simulink model "n2k_parsing"  (Simulink 7.5)
settings: Solver=FixedStepDiscrete  SolverMode=SingleTasking  StartTime=0.0  StopTime=10.0  FixedStep=0.01  RelTol=1e-3
undefined symbols (not defined in the file): enqueueNumberText, Init_Reset, initCommunications
libraries: dsPICdrivers x6, simulink x2, ecan_dspic x1
settings Model: Creator=Bryant  LastModifiedBy=Bryant
settings OptimizationCC: InlineParams=on  OptimizeModelRefInitCode=on  LifeSpan=1
settings HardwareCC: ProdBitPerInt=16  ProdEndianess=LittleEndian  ProdWordSize=16  ProdHWDeviceType=16-bit Generic
settings RTWCC: SystemTargetFile=dspic.tlc  MakeCommand=make_CreateMPLAB  TemplateMakefile=dspic_pic30_gcc.tmf  PostCodeGenCommand=dsPIC_Compile()  Description=Embedded Target for Microchip dsPIC (real-time)  ProcessScript=dspic_make_rtw_hook
settings RTWCC: CustomSource=|
  | ../../../../../ECAN_dspic/circBuffer.c
  | ../../../../../ECAN_dspic/ecanFunctions.c
  | ../../clib/uart2.c
  | extra.c
settings CodeAppCC: IgnoreCustomStorageClasses=off
settings STFCustomTargetCC: IncludeMdlTerminateFcn=off  CombineOutputUpdateFcns=on  SuppressErrorStatus=on  ERTCustomFileBanners=on  SupportContinuousTime=off  SupportNonInlinedSFcns=off  SystemTargetFile=dspic.tlc
settings ERTTargetCC: MultiwordLength=2048  ParMdlRefBuildCompliant=off  CompOptLevelCompliant=off  IncludeMdlTerminateFcn=off  SuppressErrorStatus=on  ERTFirstTimeCompliant=off  ModelStepFunctionPrototypeControlCompliant=off  CPPClassGenCompliant=off  ExtModeMexFile=ext_serial_win32_comm  InlinedParameterPlacement=NonHierarchical  ERTSrcFileBannerTemplate=dsPIC_code_template.cgt  ERTHdrFileBannerTemplate=dsPIC_code_template.cgt  ERTDataSrcFileTemplate=dsPIC_code_template.cgt  ERTDataHdrFileTemplate=dsPIC_code_template.cgt  ERTCustomFileTemplate=dsPIC_main.tlc  ConvertIfToSwitch=off
settings CustomProperty: DataType=string  Value=C:\PROGRA~1\MATLAB\R2010a\bin\win64\gmake

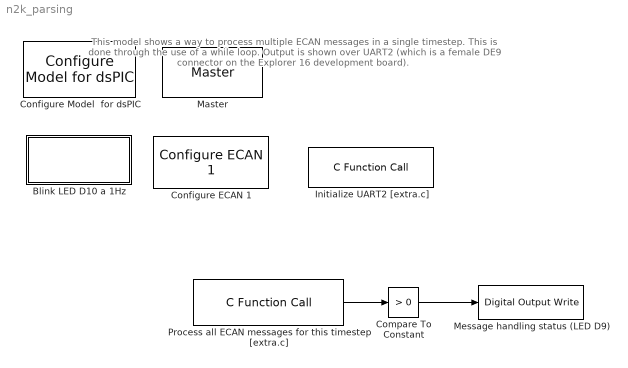
== system n2k_parsing ==
  note: This model shows a way to process multiple ECAN messages in a single timestep. This is done through the use of a while loop.
      | Output is shown over UART2 (which is a female DE9 connector on the Explorer 16 development board).
  Blink LED D10 a 1Hz : Subsystem
      mask Display: disp('blink');
  Compare To Constant : simulink/Logic and Bit Operations/Compare To Constant  SystemSampleTime=-1  relop=>  const=0  LogicOutDataTypeMode=boolean
  Configure ECAN 1 : ecan_dspic/Configure ECAN 1  SystemSampleTime=-1  frame_setting=on  mode=Normal  dma_rx_chan=2  dma_tx_chan=0  baud=250000  ps1=8  pd=5  ps2=6  sjw=4  tq=20  triple_sample=on  dma_buf_size=4 buffers  rx_bufs=[1]  tx_bufs=[0]  buf_0_tx_pri=Highest  buf_0_rte=No  buf_1_tx_pri=Highest  buf_1_rte=No  buf_2_tx_pri=Lowest  buf_2_rte=No  buf_3_tx_pri=Lowest  buf_3_rte=No  buf_4_tx_pri=Lowest  buf_4_rte=No  buf_5_tx_pri=Lowest  buf_5_rte=No  buf_6_tx_pri=Lowest  buf_6_rte=No  buf_7_tx_pri=Lowest  buf_7_rte=No  mask_0=0  mask_0_mide=Match std or ext  mask_1=0  mask_1_mide=Match std or ext  mask_2=0  mask_2_mide=Match std or ext  filters=[0]  filter_0=0  filter_0_mask=0  filter_0_exide=Match only extended  filter_0_buf=1  filter_1=hex2dec('401')  filter_1_mask=0  filter_1_exide=Match only standard  filter_1_buf=2  filter_2=hex2dec('402')  filter_2_mask=0  filter_2_exide=Match only standard  filter_2_buf=3  filter_3=0  filter_3_mask=0  filter_3_exide=Match only standard  filter_3_buf=0  filter_4=0  filter_4_mask=0  filter_4_exide=Match only standard  filter_4_buf=0  filter_5=0  filter_5_mask=0  filter_5_exide=Match only standard  filter_5_buf=0  filter_6=0  filter_6_mask=0  filter_6_exide=Match only standard  filter_6_buf=0  filter_7=0  filter_7_mask=0  filter_7_exide=Match only standard  filter_7_buf=0  filter_8=0  filter_8_mask=0  filter_8_exide=Match only standard  filter_8_buf=0  filter_9=0  filter_9_mask=<empty>  filter_9_exide=Match only standard  filter_9_buf=0  filter_10=0  filter_10_mask=0  filter_10_exide=Match only standard  filter_10_buf=0  filter_11=0  filter_11_mask=0  filter_11_exide=Match only standard  filter_11_buf=0  filter_12=0  filter_12_mask=0  filter_12_exide=Match only standard  filter_12_buf=0  filter_13=0  filter_13_mask=0  filter_13_exide=Match only standard  filter_13_buf=0  filter_14=0  filter_14_mask=0  filter_14_exide=Match only standard  filter_14_buf=0  filter_15=0  filter_15_mask=0  filter_15_exide=Match only standard  filter_15_buf=0
  Configure Model  for dsPIC : dsPICdrivers/Simulink Configuration/Configure Model  for dsPIC
  Initialize UART2 [extra.c] : dsPICdrivers/OTHERS/C Function Call  Tag=dsPIC_dsPIC_CFunctionCall  FctUpdate=None  fctName=enqueueNumberText  INPUT_SIZE=1  INPUT1=uint32  INPUT2=--  INPUT3=--  OUTPUT_SIZE=1  OUTPUT1=--  SampleTime=-1  InputType=[]  OutputType=[]  FctDeclaration=extern void enqueueNumberText();  FctCall=enqueueNumberText();  OrderingInOutPopup=None  FctStart=Start Function (Call once and only once)  FctStart_Name=initCommunications  FctStart_Declaration=inline extern void initCommunications();  FctStart_Call=initCommunications();  FctInit=None  FctInit_Name=Init_Reset  FctInit_Declaration=inline extern void Init_Reset();  FctInit_Call=Init_Reset();  PinDigitalInput=[]  PinDigitalOutput=[]  AnalogueInput=[]
  Master : dsPICdrivers/Master  Tag=dsPIC_MASTER  Priority=1  TimeStepType=Timer1  picType=33fJ256GP710  fcy=40000000  Quartz_33f=8e6  PLLActive_33f=on  fcyDesired_33f=40000000  tmr1="[8  49999  0]"  tmr1Info="Time Step : 0.01  ;   Error : 0%  PR1=49999"  tmr2345="[0  0  0  0  0  0  0  0]"  tmr2345cfg=[-1 -1 -1 -1 -1 -1 -1 -1]  IOautoConf=on  typePort="[ 0   0   0   0   0   0  10  10   0   0   0   0   0   0   0   0   0   0   0   0   0   0   0   0   0   0   0   0   0   0   0   0   0   0   0   0   0   0   0   0   0   0   0   0   0   0   0   0   0   0   0   0   0   0   0   0   0   0   0   0   0   0   0   0   0   0   0   0   0   0   0   0   0   0   0   0   0   0   0   0   0   0   0   0   0   0   0   0   0   0   0   0   0   0   0   0   0   0   0   0   0   0   0   0   0   0   0   0   0   0   0   0 ]"  TRIS="[ 65343  65535  65535  65535  65535  65535  65535 ]"  ADPCFG=12582912  MasterBusyPort=None  MasterOverloadPort=None  FOSC=Quartz (XT - HS)  ClockSwitchMonitor=Both disabled  TempProtection_33f=TEMP_ON  FPBOR=<empty>  PWRT=disable  MCLR=<empty>  ICD=ICS_PGD1  JTAGEN=JTAGEN_OFF  PowerSave=off  OverrideFcy=off  NewFcy=1e6  PR2345="[65535  65535  65535  65535  65535  65535  65535  65535]"
  Message handling status (LED D9) : dsPICdrivers/Digital I//O/Digital Output Write  Tag=dsPIC_Digital_Output  Priority=5  PORT=A  Pin=[6]  Simultaneous=off  OrderingInOutPopup=None
  Process all ECAN messages for this timestep [extra.c] : dsPICdrivers/OTHERS/C Function Call  Tag=dsPIC_dsPIC_CFunctionCall  FctUpdate=Output Function  fctName=processAllMessages  INPUT_SIZE=1  INPUT1=--  INPUT2=--  INPUT3=--  OUTPUT_SIZE=1  OUTPUT1=uint8  SampleTime=.01  InputType=[ ]  OutputType=[ 2 ]  FctDeclaration=extern uint8_T processAllMessages();  FctCall=%y1 = processAllMessages();  OrderingInOutPopup=None  FctStart=None  FctStart_Declaration=inline extern void ();  FctStart_Call=();  FctInit=None  FctInit_Name=Init_Reset  FctInit_Declaration=inline extern void Init_Reset();  FctInit_Call=Init_Reset();  PinDigitalInput=[]  PinDigitalOutput=[]  AnalogueInput=[]
  wires:
  Process all ECAN messages for this timestep [extra.c]/1 -> Compare To Constant/1
  Compare To Constant/1 -> Message handling status (LED D9)/1

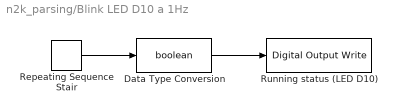
== system n2k_parsing/Blink LED D10 a 1Hz ==
  Data Type Conversion : DataTypeConversion  OutDataTypeMode=boolean  OutDataType=sfix(16)  OutScaling=2^0  OutDataTypeStr=boolean  RndMeth=Simplest
  Repeating Sequence Stair : simulink/Sources/Repeating Sequence Stair  SystemSampleTime=-1  OutValues=[1 0]  tsamp=1  OutMin=[]  OutMax=[]  OutDataTypeStr=double  OutputDataTypeScalingMode=double  OutDataType=fixdt(0,8)  ConRadixGroup=Best Precision: Vector-wise  OutScaling=2^-12
  Running status (LED D10) : dsPICdrivers/Digital I//O/Digital Output Write  Tag=dsPIC_Digital_Output  Priority=5  PORT=A  Pin=[7]  Simultaneous=off  OrderingInOutPopup=None
  wires:
  Repeating Sequence Stair/1 -> Data Type Conversion/1
  Data Type Conversion/1 -> Running status (LED D10)/1
